simulink model "fir2"  (R2015a)
settings: Solver=ode45  SolverMode=MultiTasking  StartTime=0.0  StopTime=(N-1)/Fs  MaxStep=1/Fs  MinStep=1/Fs  RelTol=1e-3  AbsTol=1/Fs
settings Model: Creator=Javi  LastModifiedBy=Javi
settings SolverCC: InitialStep=1/Fs

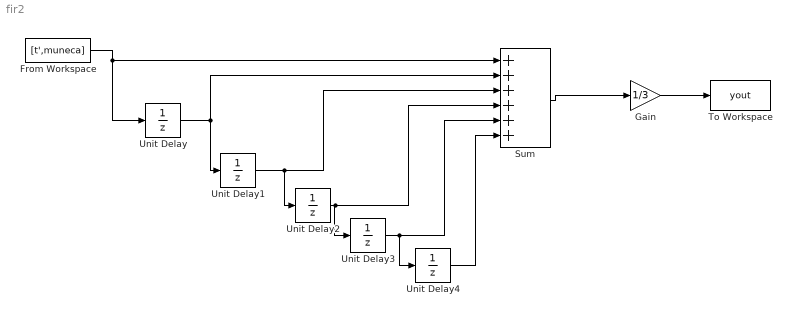
== system fir2 ==
  From Workspace : FromWorkspace  VariableName=[t',muneca]  SampleTime=0
  Gain : Gain  Gain=1/3
  Sum : Sum  Inputs=++++++
  To Workspace : ToWorkspace  VariableName=yout  SaveFormat=Timeseries  SampleTime=-1
      settings: MaxDataPoints=N
  Unit Delay{,1..4} (5 alike) : UnitDelay  SampleTime=-1
  wires:
  From Workspace/1 -> Unit Delay/1, Sum/1
  Unit Delay/1 -> Unit Delay1/1, Sum/2
  Unit Delay1/1 -> Unit Delay2/1, Sum/3
  Sum/1 -> Gain/1
  Gain/1 -> To Workspace/1
  Unit Delay2/1 -> Unit Delay3/1, Sum/4
  Unit Delay3/1 -> Unit Delay4/1, Sum/5
  Unit Delay4/1 -> Sum/6
